simulink model "Engine_Combustion_Model"  (R2016b)
settings: Solver=FixedStepAuto  StartTime=0.0  StopTime=inf  FixedStep=EngMdl.tiSimnTiStep_C  RelTol=1e-3  SampleTimeConstraint=STIndependent  EnableMultiTasking=on
undefined symbols (not defined in the file or in its folder): EngMdl
(part 1 of 2)
settings Model: Creator=m01wolf  LastModifiedBy=bunver
settings DataIOCC: SaveFormat=StructureWithTime  SaveOutput=off  DSMLogging=off  VisualizeSimOutput=off  SaveTime=off  StateSaveName=Results  SignalLoggingName=Results
settings OptimizationCC: BlockReduction=off  ConditionallyExecuteInputs=off  LifeSpan=inf
settings DebuggingCC: AllowSymbolicDim=off  SFUnexpectedBacktrackingDiag=warning  SFNoUnconditionalDefaultTransitionDiag=warning  SFExecutionAtInitializationDiag=none
settings ModelReferenceCC: ModelReferenceNumInstancesAllowed=Single  PropagateSignalLabelsOutOfModel=off
settings GRTTargetCC: TargetLangStandard=C89/C90 (ANSI)
settings ConfigComp: CovMetricSettings=dw  CovHtmlReporting=on  CovSaveCumulativeToWorkspaceVar=on  CovSaveSingleToWorkspaceVar=on  CovExternalEMLEnable=off

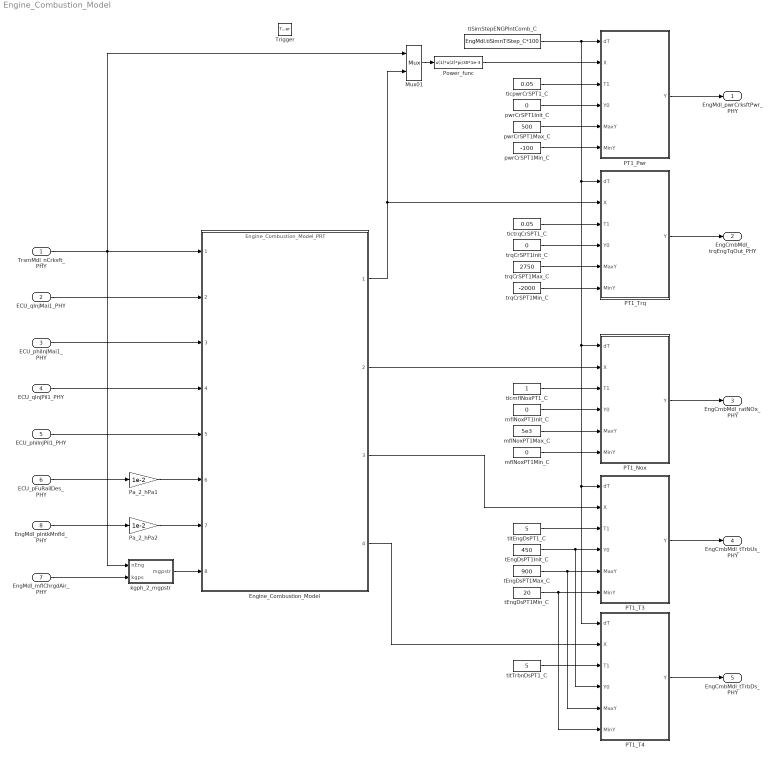
== system Engine_Combustion_Model ==
  TrsmMdl_nCrksft_PHY : Inport
  ECU_qInjMai1_PHY : Inport  Port=2
  ECU_phiInjMai1_PHY : Inport  Port=3
  ECU_qInjPil1_PHY : Inport  Port=4
  ECU_phiInjPil1_PHY : Inport  Port=5
  ECU_pFuRailDes_PHY : Inport  Port=6
  EngMdl_mflChrgdAir_PHY : Inport  Port=7
  EngMdl_pIntkMnfld_PHY : Inport  Port=8
  Trigger : TriggerPort  TriggerType=function-call  VariantControl=Variant  PortDimensions=1
  Engine_Combustion_Model : ModelReference  ModelNameDialog=Engine_Combustion_Model_PRT.slxp  ModelReferenceVersion=1.251  CopyOfModelProtected=on
  Mux01 : Mux  Inputs=2
  PT1_Nox : Subsystem
  PT1_Pwr : Subsystem
  PT1_T3 : Subsystem
  PT1_T4 : Subsystem
  PT1_Trq : Subsystem
  Pa_2_hPa1 : Gain  Gain=1e-2
  Pa_2_hPa2 : Gain  Gain=1e-2
  Power_func : Fcn  Expr=u(1)*u(2)*pi/30*1e-3
  kgph_2_mgpstr : Subsystem
  mflNoxPT1Init_C : Constant  Value=0
  mflNoxPT1Max_C : Constant  Value=5e3
  mflNoxPT1Min_C : Constant  Value=0
  pwrCrSPT1Init_C : Constant  Value=0
  pwrCrSPT1Max_C : Constant  Value=500
  pwrCrSPT1Min_C : Constant  Value=-100
  tEngDsPT1Init_C : Constant  Value=450  SampleTime=-1
  tEngDsPT1Max_C : Constant  Value=900  SampleTime=-1
  tEngDsPT1Min_C : Constant  Value=20  SampleTime=-1
  tiSimStepENGPlntComb_C : Constant  Value=EngMdl.tiSimnTiStep_C*100  SampleTime=-1
  ticmflNoxPT1_C : Constant
  ticpwrCrSPT1_C : Constant  Value=0.05
  tictrqCrSPT1_C : Constant  Value=0.05  SampleTime=-1
  titEngDsPT1_C : Constant  Value=5  SampleTime=-1
  titTrbnDsPT1_C : Constant  Value=5  SampleTime=-1
  trqCrSPT1Init_C : Constant  Value=0  SampleTime=-1
  trqCrSPT1Max_C : Constant  Value=2750  SampleTime=-1
  trqCrSPT1Min_C : Constant  Value=-2000  SampleTime=-1
  EngMdl_pwrCrksftPwr_PHY : Outport
  EngCmbMdl_trqEngTqOut_PHY : Outport  Port=2
  EngCmbMdl_ratNOx_PHY : Outport  Port=3
  EngCmbMdl_tTrbUs_PHY : Outport  Port=4
  EngCmbMdl_tTrbDs_PHY : Outport  Port=5
  wires:
  Pa_2_hPa1/1 -> Engine_Combustion_Model/6
  Pa_2_hPa2/1 -> Engine_Combustion_Model/7
  kgph_2_mgpstr/1(mgpstr) -> Engine_Combustion_Model/8
  ECU_qInjMai1_PHY/1 -> Engine_Combustion_Model/2
  ECU_phiInjMai1_PHY/1 -> Engine_Combustion_Model/3
  ECU_qInjPil1_PHY/1 -> Engine_Combustion_Model/4
  ECU_phiInjPil1_PHY/1 -> Engine_Combustion_Model/5
  ECU_pFuRailDes_PHY/1 -> Pa_2_hPa1/1
  EngMdl_mflChrgdAir_PHY/1 -> kgph_2_mgpstr/2(kgps)
  EngMdl_pIntkMnfld_PHY/1 -> Pa_2_hPa2/1
  Engine_Combustion_Model/1 -> Mux01/2, PT1_Trq/2(X)
  TrsmMdl_nCrksft_PHY/1 -> Mux01/1, Engine_Combustion_Model/1, kgph_2_mgpstr/1(nEng)
  Mux01/1 -> Power_func/1
  Engine_Combustion_Model/2 -> PT1_Nox/2(X)
  tEngDsPT1Init_C/1 -> PT1_T3/4(Y0), PT1_T4/4(Y0)
  tEngDsPT1Max_C/1 -> PT1_T3/5(MaxY), PT1_T4/5(MaxY)
  titEngDsPT1_C/1 -> PT1_T3/3(T1)
  PT1_T3/1(Y) -> EngCmbMdl_tTrbUs_PHY/1
  tEngDsPT1Min_C/1 -> PT1_T3/6(MinY), PT1_T4/6(MinY)
  Engine_Combustion_Model/3 -> PT1_T3/2(X)
  Engine_Combustion_Model/4 -> PT1_T4/2(X)
  titTrbnDsPT1_C/1 -> PT1_T4/3(T1)
  PT1_T4/1(Y) -> EngCmbMdl_tTrbDs_PHY/1
  ticmflNoxPT1_C/1 -> PT1_Nox/3(T1)
  mflNoxPT1Init_C/1 -> PT1_Nox/4(Y0)
  mflNoxPT1Max_C/1 -> PT1_Nox/5(MaxY)
  mflNoxPT1Min_C/1 -> PT1_Nox/6(MinY)
  PT1_Nox/1(Y) -> EngCmbMdl_ratNOx_PHY/1
  tictrqCrSPT1_C/1 -> PT1_Trq/3(T1)
  trqCrSPT1Init_C/1 -> PT1_Trq/4(Y0)
  trqCrSPT1Max_C/1 -> PT1_Trq/5(MaxY)
  trqCrSPT1Min_C/1 -> PT1_Trq/6(MinY)
  PT1_Trq/1(Y) -> EngCmbMdl_trqEngTqOut_PHY/1
  ticpwrCrSPT1_C/1 -> PT1_Pwr/3(T1)
  pwrCrSPT1Init_C/1 -> PT1_Pwr/4(Y0)
  pwrCrSPT1Max_C/1 -> PT1_Pwr/5(MaxY)
  pwrCrSPT1Min_C/1 -> PT1_Pwr/6(MinY)
  PT1_Pwr/1(Y) -> EngMdl_pwrCrksftPwr_PHY/1
  Power_func/1 -> PT1_Pwr/2(X)
  tiSimStepENGPlntComb_C/1 -> PT1_Trq/1(dT), PT1_Nox/1(dT), PT1_T3/1(dT), PT1_T4/1(dT), PT1_Pwr/1(dT)

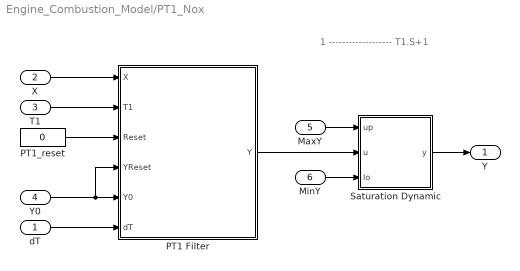
== system Engine_Combustion_Model/PT1_Nox ==
  note: 1
      | -------------------
      | T1.S+1
  dT : Inport
  X : Inport  Port=2
  T1 : Inport  Port=3
  Y0 : Inport  Port=4
  MaxY : Inport  Port=5
  MinY : Inport  Port=6
  PT1 Filter : Subsystem  mask(PT1 Filter){}
      mask help:
      | Proportional filter with first order time constant, unit gain and external reset.
      |
      | X: Input value
      | T1: Time constant of proportional filter
      | Reset: Reset status
      | YReset: Output value during reset
      | Y0: Initial value of output
      | Y: Output value
      | dT: Sample time
      mask Display:
      | color('blue');
      | fprintf('PT1\nFilter');
      | 
      | color('black');
      | port_label('input', 1, 'X');
      | port_label('input', 2, 'T1');
      | port_label('input', 3, 'Reset');
      | port_label('input', 4, 'YReset');
      | port_label('input', 5, 'Y0');
      | port_label('input', 6, 'dT');
      | port_label('output', 1, 'Y');
  PT1_reset : Constant  Value=0  SampleTime=-1
  Saturation Dynamic : Subsystem  mask(Saturation Dynamic){OutMin=[], OutMax=[], OutDataTypeStr=Inherit: Same as second input, OutputDataTypeScalingMode=Same as second input, OutDataType=fixdt(1, 16), OutScaling=2^-10, LockScale=off, RndMeth=Floor, DoSatur=off}
      mask prompts: OutMin "Simulink:masks:OutputMinimum_MP"; OutMax "Simulink:masks:OutputMaximum_MP"; OutDataTypeStr "Simulink:masks:OutputDataType_MP"; OutputDataTypeScalingMode "Simulink:masks:OutputDataTypeMode_MP"; OutDataType "Simulink:masks:OutputDataTypeegFixdt116Fixdtsingle_MP"; OutScaling "Simulink:masks:OutputScalingSlopeEg29OrSlopeBias_MP"; LockScale "Simulink:masks:LockOutputDataTypeAgainstFxpTools_MP"; RndMeth "Simulink:masks:IntegerRoundingMode_MP"; DoSatur "Simulink:masks:SaturateOnIntegerOverflow_MP"
      mask help: Simulink:masks:SaturationDynamic_MD
      mask init:
      | blkH = gcbh;
      | blkName = getfullname(blkH);
      | 
      | switch_blks = {'Switch','Switch2'}; 
      | for i = 1:length(switch_blks)
      |   set_param([blkName,'/',switch_blks{i}], ...
      |       'RndMeth', RndMeth, ...
      | 	  'DoSatur', DoSatur);
      | end
      | 
      | propBlk = [blkName, '/Data Type Propagation'];
      | 
      | if strcmp(OutputDataTypeScalingMode, 'Same as second input')
      |     set_param(propBlk, 'PropDataTypeMode', 'Inherit via propagation rule', ...
      |                        'PropScalingMode',  'Inherit via propagation rule');
      | else
      |     scaling = OutScaling;
      |     scalingMode = 'Specify via dialog';
      |     switch OutputDataTypeScalingMode
      |       case 'double'
      |         dataType = 'fixdt(''double'')';
      |       case 'single'
      |         dataType = 'fixdt(''single'')';
      |       case 'int8'
      |         dataType = 'fixdt(1,8,0)';
      |       case 'uint8'
      |         dataType = 'fixdt(0,8,0)';
      |       case 'int16'
      |         dataType = 'fixdt(1,16,0)';
      |       case 'uint16'
      |         dataType = 'fixdt(0,16,0)';
      |       case 'int32'
      |         dataType = 'fixdt(1,32,0)';
      |       case 'uint32'
      |         dataType = 'fixdt(0,32,0)';
      |       case 'Specify via dialog'
      |         dataType = OutDataType;
      |         if ~isempty(OutDataTypeStr) && isa(OutDataTypeStr,'Simulink.NumericType') 
      |           if strcmp(OutDataTypeStr.DataTypeMode, 'Fixed-point: unspecified scaling') 
      |             scalingMode = 'Obtain via best precision';
      |             range = [OutMin OutMax];
      |             range = range(~isinf(range));
      |             set_param(propBlk, 'ValuesUsedBestPrec', mat2str(range));
      |           end
      |         end
      |     end
      |     
      |     set_param(propBlk, 'PropDataTypeMode', 'Specify via dialog', ...
      |                        'PropScalingMode',  scalingMode, ...
      |                        'PropDataType',     dataType, ...
      |                        'PropScaling',      scaling);
      | end
      mask Callback OutDataTypeStr: fixptdialog(gcbh)
      mask TypeOptions OutputDataTypeScalingMode: double | single | int8 | uint8 | int16 | uint16 | int32 | uint32 | Specify via dialog | Same as second input
      mask Callback OutputDataTypeScalingMode: fixptdialog(gcbh)
      mask Callback OutDataType: fixptdialog(gcbh)
      mask TypeOptions RndMeth: Simulink:masks:Ceiling | Simulink:masks:Convergent | Simulink:masks:Floor | Simulink:masks:Nearest | Simulink:masks:Round | Simulink:masks:Simplest | Simulink:masks:Zero
  Y : Outport
  wires:
  dT/1 -> PT1 Filter/6(dT)
  MaxY/1 -> Saturation Dynamic/1(up)
  T1/1 -> PT1 Filter/2(T1)
  X/1 -> PT1 Filter/1(X)
  MinY/1 -> Saturation Dynamic/3(lo)
  Y0/1 -> PT1 Filter/5(Y0), PT1 Filter/4(YReset)
  Saturation Dynamic/1(y) -> Y/1
  PT1 Filter/1(Y) -> Saturation Dynamic/2(u)
  PT1_reset/1 -> PT1 Filter/3(Reset)

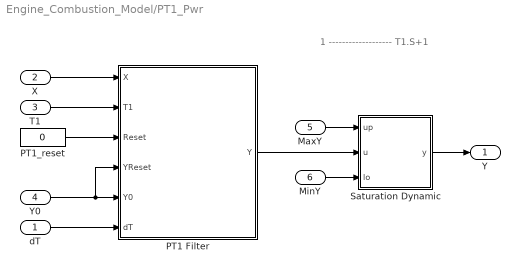
== system Engine_Combustion_Model/PT1_Pwr ==
  note: 1
      | -------------------
      | T1.S+1
  dT : Inport
  X : Inport  Port=2
  T1 : Inport  Port=3
  Y0 : Inport  Port=4
  MaxY : Inport  Port=5
  MinY : Inport  Port=6
  PT1 Filter : Subsystem  mask(PT1 Filter){}
      mask help:
      | Proportional filter with first order time constant, unit gain and external reset.
      |
      | X: Input value
      | T1: Time constant of proportional filter
      | Reset: Reset status
      | YReset: Output value during reset
      | Y0: Initial value of output
      | Y: Output value
      | dT: Sample time
      mask Display:
      | color('blue');
      | fprintf('PT1\nFilter');
      | 
      | color('black');
      | port_label('input', 1, 'X');
      | port_label('input', 2, 'T1');
      | port_label('input', 3, 'Reset');
      | port_label('input', 4, 'YReset');
      | port_label('input', 5, 'Y0');
      | port_label('input', 6, 'dT');
      | port_label('output', 1, 'Y');
  PT1_reset : Constant  Value=0  SampleTime=-1
  Saturation Dynamic : Subsystem  mask(Saturation Dynamic){OutMin=[], OutMax=[], OutDataTypeStr=Inherit: Same as second input, OutputDataTypeScalingMode=Same as second input, OutDataType=fixdt(1, 16), OutScaling=2^-10, LockScale=off, RndMeth=Floor, DoSatur=off}
      mask prompts: OutMin "Simulink:masks:OutputMinimum_MP"; OutMax "Simulink:masks:OutputMaximum_MP"; OutDataTypeStr "Simulink:masks:OutputDataType_MP"; OutputDataTypeScalingMode "Simulink:masks:OutputDataTypeMode_MP"; OutDataType "Simulink:masks:OutputDataTypeegFixdt116Fixdtsingle_MP"; OutScaling "Simulink:masks:OutputScalingSlopeEg29OrSlopeBias_MP"; LockScale "Simulink:masks:LockOutputDataTypeAgainstFxpTools_MP"; RndMeth "Simulink:masks:IntegerRoundingMode_MP"; DoSatur "Simulink:masks:SaturateOnIntegerOverflow_MP"
      mask help: Simulink:masks:SaturationDynamic_MD
      mask init: same as Engine_Combustion_Model/PT1_Nox/Saturation Dynamic
      mask Callback OutDataTypeStr: fixptdialog(gcbh)
      mask TypeOptions OutputDataTypeScalingMode: double | single | int8 | uint8 | int16 | uint16 | int32 | uint32 | Specify via dialog | Same as second input
      mask Callback OutputDataTypeScalingMode: fixptdialog(gcbh)
      mask Callback OutDataType: fixptdialog(gcbh)
      mask TypeOptions RndMeth: Simulink:masks:Ceiling | Simulink:masks:Convergent | Simulink:masks:Floor | Simulink:masks:Nearest | Simulink:masks:Round | Simulink:masks:Simplest | Simulink:masks:Zero
  Y : Outport
  wires:
  dT/1 -> PT1 Filter/6(dT)
  MaxY/1 -> Saturation Dynamic/1(up)
  T1/1 -> PT1 Filter/2(T1)
  X/1 -> PT1 Filter/1(X)
  MinY/1 -> Saturation Dynamic/3(lo)
  Y0/1 -> PT1 Filter/5(Y0), PT1 Filter/4(YReset)
  Saturation Dynamic/1(y) -> Y/1
  PT1 Filter/1(Y) -> Saturation Dynamic/2(u)
  PT1_reset/1 -> PT1 Filter/3(Reset)

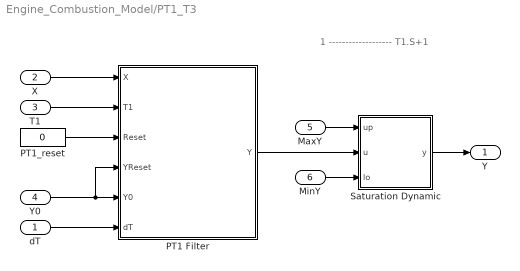
== system Engine_Combustion_Model/PT1_T3 ==
  note: 1
      | -------------------
      | T1.S+1
  dT : Inport
  X : Inport  Port=2
  T1 : Inport  Port=3
  Y0 : Inport  Port=4
  MaxY : Inport  Port=5
  MinY : Inport  Port=6
  PT1 Filter : Subsystem  mask(PT1 Filter){}
      mask help:
      | Proportional filter with first order time constant, unit gain and external reset.
      |
      | X: Input value
      | T1: Time constant of proportional filter
      | Reset: Reset status
      | YReset: Output value during reset
      | Y0: Initial value of output
      | Y: Output value
      | dT: Sample time
      mask Display:
      | color('blue');
      | fprintf('PT1\nFilter');
      | 
      | color('black');
      | port_label('input', 1, 'X');
      | port_label('input', 2, 'T1');
      | port_label('input', 3, 'Reset');
      | port_label('input', 4, 'YReset');
      | port_label('input', 5, 'Y0');
      | port_label('input', 6, 'dT');
      | port_label('output', 1, 'Y');
  PT1_reset : Constant  Value=0  SampleTime=-1
  Saturation Dynamic : Subsystem  mask(Saturation Dynamic){OutMin=[], OutMax=[], OutDataTypeStr=Inherit: Same as second input, OutputDataTypeScalingMode=Same as second input, OutDataType=fixdt(1, 16), OutScaling=2^-10, LockScale=off, RndMeth=Floor, DoSatur=off}
      mask prompts: OutMin "Simulink:masks:OutputMinimum_MP"; OutMax "Simulink:masks:OutputMaximum_MP"; OutDataTypeStr "Simulink:masks:OutputDataType_MP"; OutputDataTypeScalingMode "Simulink:masks:OutputDataTypeMode_MP"; OutDataType "Simulink:masks:OutputDataTypeegFixdt116Fixdtsingle_MP"; OutScaling "Simulink:masks:OutputScalingSlopeEg29OrSlopeBias_MP"; LockScale "Simulink:masks:LockOutputDataTypeAgainstFxpTools_MP"; RndMeth "Simulink:masks:IntegerRoundingMode_MP"; DoSatur "Simulink:masks:SaturateOnIntegerOverflow_MP"
      mask help: Simulink:masks:SaturationDynamic_MD
      mask init: same as Engine_Combustion_Model/PT1_Nox/Saturation Dynamic
      mask Callback OutDataTypeStr: fixptdialog(gcbh)
      mask TypeOptions OutputDataTypeScalingMode: double | single | int8 | uint8 | int16 | uint16 | int32 | uint32 | Specify via dialog | Same as second input
      mask Callback OutputDataTypeScalingMode: fixptdialog(gcbh)
      mask Callback OutDataType: fixptdialog(gcbh)
      mask TypeOptions RndMeth: Simulink:masks:Ceiling | Simulink:masks:Convergent | Simulink:masks:Floor | Simulink:masks:Nearest | Simulink:masks:Round | Simulink:masks:Simplest | Simulink:masks:Zero
  Y : Outport
  wires:
  PT1_reset/1 -> PT1 Filter/3(Reset)
  PT1 Filter/1(Y) -> Saturation Dynamic/2(u)
  Saturation Dynamic/1(y) -> Y/1
  Y0/1 -> PT1 Filter/4(YReset), PT1 Filter/5(Y0)
  MinY/1 -> Saturation Dynamic/3(lo)
  X/1 -> PT1 Filter/1(X)
  T1/1 -> PT1 Filter/2(T1)
  MaxY/1 -> Saturation Dynamic/1(up)
  dT/1 -> PT1 Filter/6(dT)

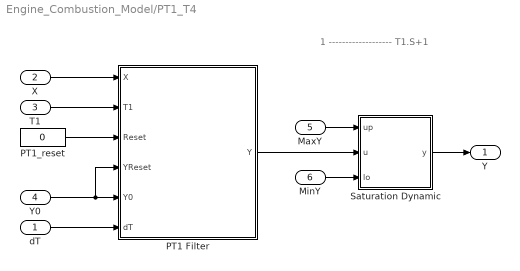
== system Engine_Combustion_Model/PT1_T4 ==
  note: 1
      | -------------------
      | T1.S+1
  dT : Inport
  X : Inport  Port=2
  T1 : Inport  Port=3
  Y0 : Inport  Port=4
  MaxY : Inport  Port=5
  MinY : Inport  Port=6
  PT1 Filter : Subsystem  mask(PT1 Filter){}
      mask help:
      | Proportional filter with first order time constant, unit gain and external reset.
      |
      | X: Input value
      | T1: Time constant of proportional filter
      | Reset: Reset status
      | YReset: Output value during reset
      | Y0: Initial value of output
      | Y: Output value
      | dT: Sample time
      mask Display:
      | color('blue');
      | fprintf('PT1\nFilter');
      | 
      | color('black');
      | port_label('input', 1, 'X');
      | port_label('input', 2, 'T1');
      | port_label('input', 3, 'Reset');
      | port_label('input', 4, 'YReset');
      | port_label('input', 5, 'Y0');
      | port_label('input', 6, 'dT');
      | port_label('output', 1, 'Y');
  PT1_reset : Constant  Value=0  SampleTime=-1
  Saturation Dynamic : Subsystem  mask(Saturation Dynamic){OutMin=[], OutMax=[], OutDataTypeStr=Inherit: Same as second input, OutputDataTypeScalingMode=Same as second input, OutDataType=fixdt(1, 16), OutScaling=2^-10, LockScale=off, RndMeth=Floor, DoSatur=off}
      mask prompts: OutMin "Simulink:masks:OutputMinimum_MP"; OutMax "Simulink:masks:OutputMaximum_MP"; OutDataTypeStr "Simulink:masks:OutputDataType_MP"; OutputDataTypeScalingMode "Simulink:masks:OutputDataTypeMode_MP"; OutDataType "Simulink:masks:OutputDataTypeegFixdt116Fixdtsingle_MP"; OutScaling "Simulink:masks:OutputScalingSlopeEg29OrSlopeBias_MP"; LockScale "Simulink:masks:LockOutputDataTypeAgainstFxpTools_MP"; RndMeth "Simulink:masks:IntegerRoundingMode_MP"; DoSatur "Simulink:masks:SaturateOnIntegerOverflow_MP"
      mask help: Simulink:masks:SaturationDynamic_MD
      mask init: same as Engine_Combustion_Model/PT1_Nox/Saturation Dynamic
      mask Callback OutDataTypeStr: fixptdialog(gcbh)
      mask TypeOptions OutputDataTypeScalingMode: double | single | int8 | uint8 | int16 | uint16 | int32 | uint32 | Specify via dialog | Same as second input
      mask Callback OutputDataTypeScalingMode: fixptdialog(gcbh)
      mask Callback OutDataType: fixptdialog(gcbh)
      mask TypeOptions RndMeth: Simulink:masks:Ceiling | Simulink:masks:Convergent | Simulink:masks:Floor | Simulink:masks:Nearest | Simulink:masks:Round | Simulink:masks:Simplest | Simulink:masks:Zero
  Y : Outport
  wires:
  dT/1 -> PT1 Filter/6(dT)
  MaxY/1 -> Saturation Dynamic/1(up)
  T1/1 -> PT1 Filter/2(T1)
  X/1 -> PT1 Filter/1(X)
  MinY/1 -> Saturation Dynamic/3(lo)
  Y0/1 -> PT1 Filter/5(Y0), PT1 Filter/4(YReset)
  Saturation Dynamic/1(y) -> Y/1
  PT1 Filter/1(Y) -> Saturation Dynamic/2(u)
  PT1_reset/1 -> PT1 Filter/3(Reset)

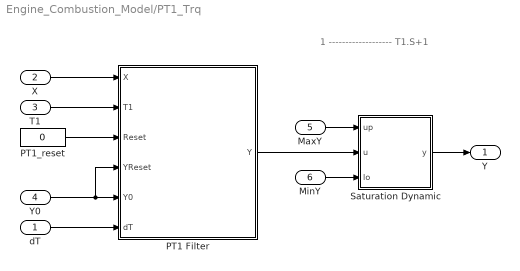
== system Engine_Combustion_Model/PT1_Trq ==
  note: 1
      | -------------------
      | T1.S+1
  dT : Inport
  X : Inport  Port=2
  T1 : Inport  Port=3
  Y0 : Inport  Port=4
  MaxY : Inport  Port=5
  MinY : Inport  Port=6
  PT1 Filter : Subsystem  mask(PT1 Filter){}
      mask help:
      | Proportional filter with first order time constant, unit gain and external reset.
      |
      | X: Input value
      | T1: Time constant of proportional filter
      | Reset: Reset status
      | YReset: Output value during reset
      | Y0: Initial value of output
      | Y: Output value
      | dT: Sample time
      mask Display:
      | color('blue');
      | fprintf('PT1\nFilter');
      | 
      | color('black');
      | port_label('input', 1, 'X');
      | port_label('input', 2, 'T1');
      | port_label('input', 3, 'Reset');
      | port_label('input', 4, 'YReset');
      | port_label('input', 5, 'Y0');
      | port_label('input', 6, 'dT');
      | port_label('output', 1, 'Y');
  PT1_reset : Constant  Value=0  SampleTime=-1
  Saturation Dynamic : Subsystem  mask(Saturation Dynamic){OutMin=[], OutMax=[], OutDataTypeStr=Inherit: Same as second input, OutputDataTypeScalingMode=Same as second input, OutDataType=fixdt(1, 16), OutScaling=2^-10, LockScale=off, RndMeth=Floor, DoSatur=off}
      mask prompts: OutMin "Simulink:masks:OutputMinimum_MP"; OutMax "Simulink:masks:OutputMaximum_MP"; OutDataTypeStr "Simulink:masks:OutputDataType_MP"; OutputDataTypeScalingMode "Simulink:masks:OutputDataTypeMode_MP"; OutDataType "Simulink:masks:OutputDataTypeegFixdt116Fixdtsingle_MP"; OutScaling "Simulink:masks:OutputScalingSlopeEg29OrSlopeBias_MP"; LockScale "Simulink:masks:LockOutputDataTypeAgainstFxpTools_MP"; RndMeth "Simulink:masks:IntegerRoundingMode_MP"; DoSatur "Simulink:masks:SaturateOnIntegerOverflow_MP"
      mask help: Simulink:masks:SaturationDynamic_MD
      mask init: same as Engine_Combustion_Model/PT1_Nox/Saturation Dynamic
      mask Callback OutDataTypeStr: fixptdialog(gcbh)
      mask TypeOptions OutputDataTypeScalingMode: double | single | int8 | uint8 | int16 | uint16 | int32 | uint32 | Specify via dialog | Same as second input
      mask Callback OutputDataTypeScalingMode: fixptdialog(gcbh)
      mask Callback OutDataType: fixptdialog(gcbh)
      mask TypeOptions RndMeth: Simulink:masks:Ceiling | Simulink:masks:Convergent | Simulink:masks:Floor | Simulink:masks:Nearest | Simulink:masks:Round | Simulink:masks:Simplest | Simulink:masks:Zero
  Y : Outport
  wires:
  PT1_reset/1 -> PT1 Filter/3(Reset)
  PT1 Filter/1(Y) -> Saturation Dynamic/2(u)
  Saturation Dynamic/1(y) -> Y/1
  Y0/1 -> PT1 Filter/4(YReset), PT1 Filter/5(Y0)
  MinY/1 -> Saturation Dynamic/3(lo)
  X/1 -> PT1 Filter/1(X)
  T1/1 -> PT1 Filter/2(T1)
  MaxY/1 -> Saturation Dynamic/1(up)
  dT/1 -> PT1 Filter/6(dT)

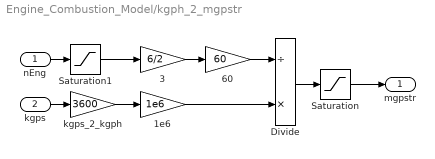
== system Engine_Combustion_Model/kgph_2_mgpstr ==
  nEng : Inport
  kgps : Inport  Port=2
  1e6 : Gain  Gain=1e6
  3 : Gain  Gain=6/2
  60 : Gain  Gain=60
  Divide : Product  Inputs=/*
  Saturation : Saturate  UpperLimit=inf  LowerLimit=0
  Saturation1 : Saturate  UpperLimit=inf  LowerLimit=300
  kgps_2_kgph : Gain  Gain=3600
  mgpstr : Outport
  wires:
  Saturation1/1 -> 3/1
  Divide/1 -> Saturation/1
  nEng/1 -> Saturation1/1
  kgps/1 -> kgps_2_kgph/1
  Saturation/1 -> mgpstr/1
  kgps_2_kgph/1 -> 1e6/1
  1e6/1 -> Divide/2
  3/1 -> 60/1
  60/1 -> Divide/1

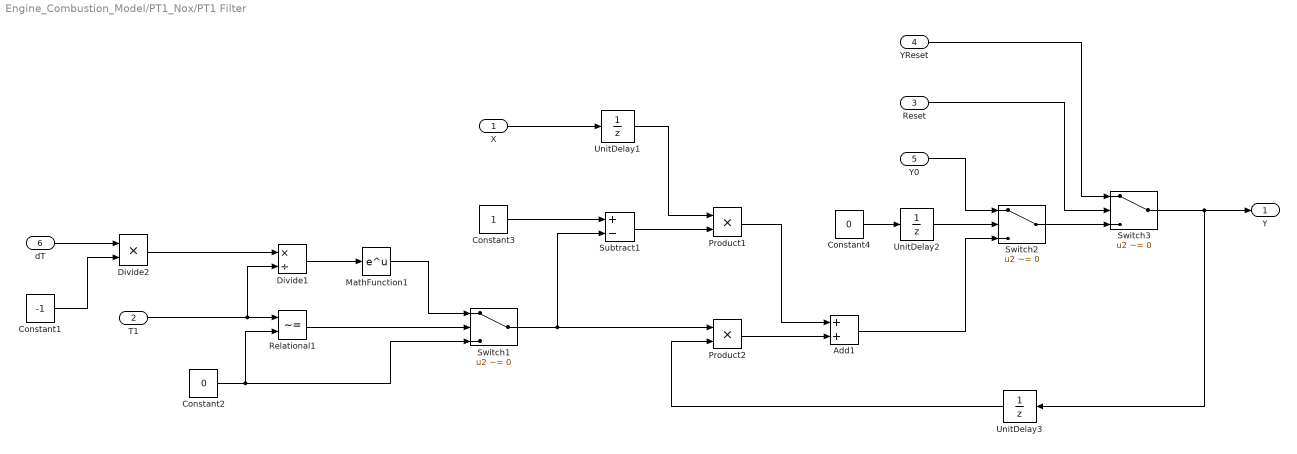
== system Engine_Combustion_Model/PT1_Nox/PT1 Filter ==
  X : Inport
  T1 : Inport  Port=2
  Reset : Inport  Port=3
  YReset : Inport  Port=4
  Y0 : Inport  Port=5
  dT : Inport  Port=6
  Add1 : Sum
  Constant1 : Constant  Value=-1
  Constant2 : Constant  Value=0
  Constant3 : Constant
  Constant4 : Constant  Value=0
  Divide1 : Product  Inputs=*/
  Divide2 : Product  Inputs=**
  MathFunction1 : Math  SaturateOnIntegerOverflow=on
  Product1 : Product  RndMeth=Zero
  Product2 : Product  RndMeth=Zero
  Relational1 : RelationalOperator  Operator=~=  OutDataTypeStr=boolean  RndMeth=Nearest
  Subtract1 : Sum  Inputs=+-
  Switch1 : Switch  Criteria=u2 ~= 0
  Switch2 : Switch  Criteria=u2 ~= 0
  Switch3 : Switch  Criteria=u2 ~= 0
  UnitDelay1 : UnitDelay  SampleTime=-1
  UnitDelay2 : UnitDelay  InitialCondition=1  SampleTime=-1
  UnitDelay3 : UnitDelay  SampleTime=-1
  Y : Outport
  wires:
  dT/1 -> Divide2/1
  Constant2/1 -> Relational1/2, Switch1/3
  MathFunction1/1 -> Switch1/1
  Relational1/1 -> Switch1/2
  Switch2/1 -> Switch3/3
  Add1/1 -> Switch2/3
  Switch3/1 -> Y/1, UnitDelay3/1
  Y0/1 -> Switch2/1
  UnitDelay2/1 -> Switch2/2
  Constant4/1 -> UnitDelay2/1
  YReset/1 -> Switch3/1
  Reset/1 -> Switch3/2
  UnitDelay3/1 -> Product2/2
  Switch1/1 -> Product2/1, Subtract1/2
  Product2/1 -> Add1/2
  Product1/1 -> Add1/1
  Subtract1/1 -> Product1/2
  UnitDelay1/1 -> Product1/1
  X/1 -> UnitDelay1/1
  Constant3/1 -> Subtract1/1
  Divide1/1 -> MathFunction1/1
  Divide2/1 -> Divide1/1
  T1/1 -> Relational1/1, Divide1/2
  Constant1/1 -> Divide2/2

== system Engine_Combustion_Model/PT1_Nox/Saturation Dynamic ==
  up : Inport
  u : Inport  Port=2
  lo : Inport  Port=3
  Data Type Duplicate : DataTypeDuplicate  DisableCoverage=on
  Data Type Propagation : S-Function  FunctionName=sfix_dtprop  Parameters=14,PropDataTypeMode,(getdatatypespecs(PropDataType,PropScaling,DblOver,0, 0, PropDataTypeMode, PropScalingMode)),IfRefDouble,IfRefSingle,IsSigned,NumBitsBase,NumBitsMult,NumBitsAdd,(sort(reshape(round(NumBitsAllowFinal), prod(size(NumBitsAllowFinal)),1))),PropScalingMode,ValuesUsedBestPrec,SlopeBase,SlopeMult,SlopeAdd,BiasBase,BiasMult,BiasAdd,DblOver  SFunctionDeploymentMode=off  EnableBusSupport=off  mask(Data Type Propagation){PropDataTypeMode=Inherit via propagation rule, PropDataType=fixdt(1, 16), IfRefDouble=double, IfRefSingle=single, IsSigned=IsSigned1, NumBitsBase=NumBits1, NumBitsMult=1, NumBitsAdd=0, NumBitsAllowFinal=1:128, PropScalingMode=Inherit via propagation rule, PropScaling=2^-10, ValuesUsedBestPrec=[5 -7], SlopeBase=Slope1, SlopeMult=1, SlopeAdd=0, BiasBase=Bias1, BiasMult=1, BiasAdd=0}
      mask prompts: PropDataTypeMode "Simulink:masks:x1PropagatedDataType_MP"; PropDataType "Simulink:masks:x11PropagatedDataTypeegFixdt116Fixdtsingle_MP"; IfRefDouble "Simulink:masks:x11IfAnyReferenceInputIsDoubleOutputIs_MP"; IfRefSingle "Simulink:masks:x12IfAnyReferenceInputIsSingleOutputIs_MP"; IsSigned "Simulink:masks:x13IsSigned_MP"; NumBitsBase "Simulink:masks:x141NumberofBitsBase_MP"; NumBitsMult "Simulink:masks:x142NumberofBitsMultiplicativeAdjustment_MP"; NumBitsAdd "Simulink:masks:x143NumberofBitsAdditiveAdjustment_MP"; NumBitsAllowFinal "Simulink:masks:x144NumberofBitsAllowableFinalValues_MP"; PropScalingMode "Simulink:masks:x2PropagatedScaling_MP"; PropScaling "Simulink:masks:x21PropagatedScalingSlopeEg29OrSlopeBiasEg1253_MP"; ValuesUsedBestPrec "Simulink:masks:x21ValuesUsedToDetermineBestPrecisionScaling_MP"; SlopeBase "Simulink:masks:x211SlopeBase_MP"; SlopeMult "Simulink:masks:x212SlopeMultiplicativeAdjustment_MP"; SlopeAdd "Simulink:masks:x213SlopeAdditiveAdjustment_MP"; BiasBase "Simulink:masks:x221BiasBase_MP"; BiasMult "Simulink:masks:x222BiasMultiplicativeAdjustment_MP"; BiasAdd "Simulink:masks:x223BiasAdditiveAdjustment_MP"
      mask help: Simulink:masks:DataTypePropagation_MD
      mask init:
      | DblOver = 0;
      mask TypeOptions PropDataTypeMode: Simulink:masks:SpecifyViaDialog | Simulink:masks:InheritViaPropagationRule
      mask Callback PropDataTypeMode: fixptdialog(gcbh)
      mask Callback PropDataType: fixptdialog(gcbh)
      mask TypeOptions IfRefDouble: Simulink:masks:double | Simulink:masks:single
      mask TypeOptions IfRefSingle: Simulink:masks:double | Simulink:masks:single
      mask TypeOptions IsSigned: Simulink:masks:IsSigned1 | Simulink:masks:IsSigned2 | Simulink:masks:IsSigned1OrIsSigned2 | Simulink:masks:TRUE | Simulink:masks:FALSE
      mask TypeOptions NumBitsBase: NumBits1 | NumBits2 | max([NumBits1 NumBits2]) | min([NumBits1 NumBits2]) | NumBits1+NumBits2
      mask TypeOptions PropScalingMode: Simulink:masks:SpecifyViaDialog | Simulink:masks:InheritViaPropagationRule | Simulink:masks:ObtainViaBestPrecision
      mask Callback PropScalingMode: fixptdialog(gcbh)
      mask TypeOptions SlopeBase: Slope1 | Slope2 | max([Slope1 Slope2]) | min([Slope1 Slope2]) | Slope1*Slope2 | Slope1/Slope2 | PosRange1 | PosRange2 | max([PosRange1 PosRange2]) | min([PosRange1 PosRange2]) | PosRange1*PosRange2 | PosRange1/PosRange2
      mask TypeOptions BiasBase: Bias1 | Bias2 | max([Bias1 Bias2]) | min([Bias1 Bias2]) | Bias1*Bias2 | Bias1/Bias2 | Bias1+Bias2 | Bias1-Bias2
      mask Display:
      | port_label('Input',1,'Ref1');
      | port_label('Input',2,'Ref2');
      | port_label('Input',3,'Prop');
  LowerRelop1 : RelationalOperator  DisableCoverage=on  Operator=>  OutDataTypeStr=boolean  RndMeth=Nearest
  Switch : Switch  Criteria=u2 ~= 0  OutDataTypeStr=Inherit: Inherit via back propagation  ZeroCross=off
  Switch2 : Switch  Criteria=u2 ~= 0  OutMin=OutMin  OutMax=OutMax  OutDataTypeStr=Inherit: Inherit via back propagation  ZeroCross=off
  UpperRelop : RelationalOperator  DisableCoverage=on  Operator=<  OutDataTypeStr=boolean  RndMeth=Nearest
  y : Outport  OutMin=OutMin  OutMax=OutMax
  wires:
  up/1 -> Switch2/1, LowerRelop1/2
  u/1 -> Data Type Propagation/2, Data Type Propagation/1, LowerRelop1/1, Switch/3, UpperRelop/1
  lo/1 -> Switch/1, UpperRelop/2
  Switch/1 -> Data Type Duplicate/2, Switch2/3, Data Type Propagation/3
  Switch2/1 -> Data Type Duplicate/1, y/1
  LowerRelop1/1 -> Switch2/2
  UpperRelop/1 -> Switch/2

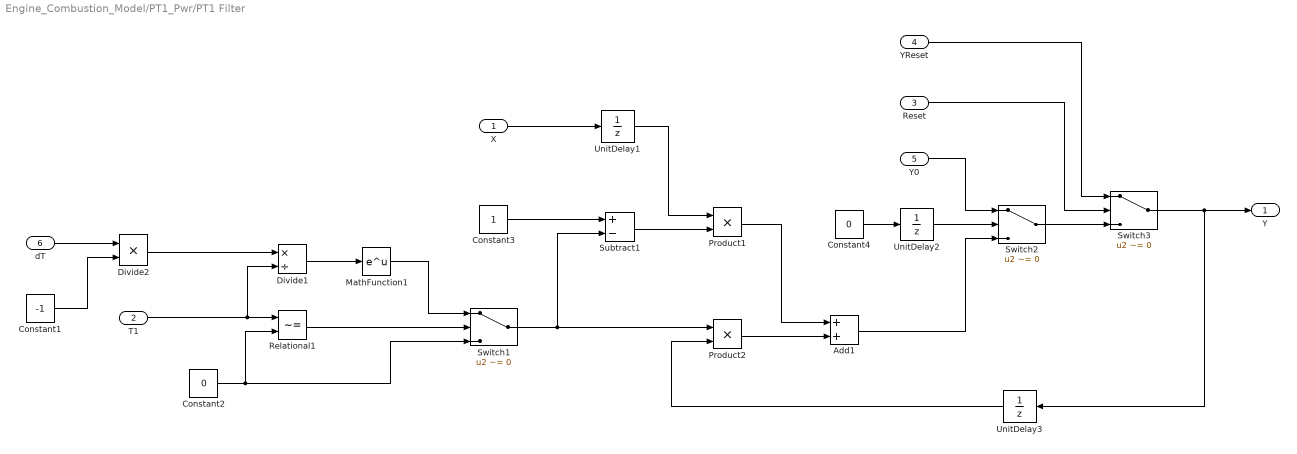
== system Engine_Combustion_Model/PT1_Pwr/PT1 Filter ==
  X : Inport
  T1 : Inport  Port=2
  Reset : Inport  Port=3
  YReset : Inport  Port=4
  Y0 : Inport  Port=5
  dT : Inport  Port=6
  Add1 : Sum
  Constant1 : Constant  Value=-1
  Constant2 : Constant  Value=0
  Constant3 : Constant
  Constant4 : Constant  Value=0
  Divide1 : Product  Inputs=*/
  Divide2 : Product  Inputs=**
  MathFunction1 : Math  SaturateOnIntegerOverflow=on
  Product1 : Product  RndMeth=Zero
  Product2 : Product  RndMeth=Zero
  Relational1 : RelationalOperator  Operator=~=  OutDataTypeStr=boolean  RndMeth=Nearest
  Subtract1 : Sum  Inputs=+-
  Switch1 : Switch  Criteria=u2 ~= 0
  Switch2 : Switch  Criteria=u2 ~= 0
  Switch3 : Switch  Criteria=u2 ~= 0
  UnitDelay1 : UnitDelay  SampleTime=-1
  UnitDelay2 : UnitDelay  InitialCondition=1  SampleTime=-1
  UnitDelay3 : UnitDelay  SampleTime=-1
  Y : Outport
  wires:
  dT/1 -> Divide2/1
  Constant2/1 -> Relational1/2, Switch1/3
  MathFunction1/1 -> Switch1/1
  Relational1/1 -> Switch1/2
  Switch2/1 -> Switch3/3
  Add1/1 -> Switch2/3
  Switch3/1 -> Y/1, UnitDelay3/1
  Y0/1 -> Switch2/1
  UnitDelay2/1 -> Switch2/2
  Constant4/1 -> UnitDelay2/1
  YReset/1 -> Switch3/1
  Reset/1 -> Switch3/2
  UnitDelay3/1 -> Product2/2
  Switch1/1 -> Product2/1, Subtract1/2
  Product2/1 -> Add1/2
  Product1/1 -> Add1/1
  Subtract1/1 -> Product1/2
  UnitDelay1/1 -> Product1/1
  X/1 -> UnitDelay1/1
  Constant3/1 -> Subtract1/1
  Divide1/1 -> MathFunction1/1
  Divide2/1 -> Divide1/1
  T1/1 -> Relational1/1, Divide1/2
  Constant1/1 -> Divide2/2

== system Engine_Combustion_Model/PT1_Pwr/Saturation Dynamic ==
  up : Inport
  u : Inport  Port=2
  lo : Inport  Port=3
  Data Type Duplicate : DataTypeDuplicate  DisableCoverage=on
  Data Type Propagation : S-Function  FunctionName=sfix_dtprop  Parameters=14,PropDataTypeMode,(getdatatypespecs(PropDataType,PropScaling,DblOver,0, 0, PropDataTypeMode, PropScalingMode)),IfRefDouble,IfRefSingle,IsSigned,NumBitsBase,NumBitsMult,NumBitsAdd,(sort(reshape(round(NumBitsAllowFinal), prod(size(NumBitsAllowFinal)),1))),PropScalingMode,ValuesUsedBestPrec,SlopeBase,SlopeMult,SlopeAdd,BiasBase,BiasMult,BiasAdd,DblOver  SFunctionDeploymentMode=off  EnableBusSupport=off  mask(Data Type Propagation){PropDataTypeMode=Inherit via propagation rule, PropDataType=fixdt(1, 16), IfRefDouble=double, IfRefSingle=single, IsSigned=IsSigned1, NumBitsBase=NumBits1, NumBitsMult=1, NumBitsAdd=0, NumBitsAllowFinal=1:128, PropScalingMode=Inherit via propagation rule, PropScaling=2^-10, ValuesUsedBestPrec=[5 -7], SlopeBase=Slope1, SlopeMult=1, SlopeAdd=0, BiasBase=Bias1, BiasMult=1, BiasAdd=0}
      mask prompts: PropDataTypeMode "Simulink:masks:x1PropagatedDataType_MP"; PropDataType "Simulink:masks:x11PropagatedDataTypeegFixdt116Fixdtsingle_MP"; IfRefDouble "Simulink:masks:x11IfAnyReferenceInputIsDoubleOutputIs_MP"; IfRefSingle "Simulink:masks:x12IfAnyReferenceInputIsSingleOutputIs_MP"; IsSigned "Simulink:masks:x13IsSigned_MP"; NumBitsBase "Simulink:masks:x141NumberofBitsBase_MP"; NumBitsMult "Simulink:masks:x142NumberofBitsMultiplicativeAdjustment_MP"; NumBitsAdd "Simulink:masks:x143NumberofBitsAdditiveAdjustment_MP"; NumBitsAllowFinal "Simulink:masks:x144NumberofBitsAllowableFinalValues_MP"; PropScalingMode "Simulink:masks:x2PropagatedScaling_MP"; PropScaling "Simulink:masks:x21PropagatedScalingSlopeEg29OrSlopeBiasEg1253_MP"; ValuesUsedBestPrec "Simulink:masks:x21ValuesUsedToDetermineBestPrecisionScaling_MP"; SlopeBase "Simulink:masks:x211SlopeBase_MP"; SlopeMult "Simulink:masks:x212SlopeMultiplicativeAdjustment_MP"; SlopeAdd "Simulink:masks:x213SlopeAdditiveAdjustment_MP"; BiasBase "Simulink:masks:x221BiasBase_MP"; BiasMult "Simulink:masks:x222BiasMultiplicativeAdjustment_MP"; BiasAdd "Simulink:masks:x223BiasAdditiveAdjustment_MP"
      mask help: Simulink:masks:DataTypePropagation_MD
      mask init:
      | DblOver = 0;
      mask TypeOptions PropDataTypeMode: Simulink:masks:SpecifyViaDialog | Simulink:masks:InheritViaPropagationRule
      mask Callback PropDataTypeMode: fixptdialog(gcbh)
      mask Callback PropDataType: fixptdialog(gcbh)
      mask TypeOptions IfRefDouble: Simulink:masks:double | Simulink:masks:single
      mask TypeOptions IfRefSingle: Simulink:masks:double | Simulink:masks:single
      mask TypeOptions IsSigned: Simulink:masks:IsSigned1 | Simulink:masks:IsSigned2 | Simulink:masks:IsSigned1OrIsSigned2 | Simulink:masks:TRUE | Simulink:masks:FALSE
      mask TypeOptions NumBitsBase: NumBits1 | NumBits2 | max([NumBits1 NumBits2]) | min([NumBits1 NumBits2]) | NumBits1+NumBits2
      mask TypeOptions PropScalingMode: Simulink:masks:SpecifyViaDialog | Simulink:masks:InheritViaPropagationRule | Simulink:masks:ObtainViaBestPrecision
      mask Callback PropScalingMode: fixptdialog(gcbh)
      mask TypeOptions SlopeBase: Slope1 | Slope2 | max([Slope1 Slope2]) | min([Slope1 Slope2]) | Slope1*Slope2 | Slope1/Slope2 | PosRange1 | PosRange2 | max([PosRange1 PosRange2]) | min([PosRange1 PosRange2]) | PosRange1*PosRange2 | PosRange1/PosRange2
      mask TypeOptions BiasBase: Bias1 | Bias2 | max([Bias1 Bias2]) | min([Bias1 Bias2]) | Bias1*Bias2 | Bias1/Bias2 | Bias1+Bias2 | Bias1-Bias2
      mask Display:
      | port_label('Input',1,'Ref1');
      | port_label('Input',2,'Ref2');
      | port_label('Input',3,'Prop');
  LowerRelop1 : RelationalOperator  DisableCoverage=on  Operator=>  OutDataTypeStr=boolean  RndMeth=Nearest
  Switch : Switch  Criteria=u2 ~= 0  OutDataTypeStr=Inherit: Inherit via back propagation  ZeroCross=off
  Switch2 : Switch  Criteria=u2 ~= 0  OutMin=OutMin  OutMax=OutMax  OutDataTypeStr=Inherit: Inherit via back propagation  ZeroCross=off
  UpperRelop : RelationalOperator  DisableCoverage=on  Operator=<  OutDataTypeStr=boolean  RndMeth=Nearest
  y : Outport  OutMin=OutMin  OutMax=OutMax
  wires:
  up/1 -> Switch2/1, LowerRelop1/2
  u/1 -> Data Type Propagation/2, Data Type Propagation/1, LowerRelop1/1, Switch/3, UpperRelop/1
  lo/1 -> Switch/1, UpperRelop/2
  Switch/1 -> Data Type Duplicate/2, Switch2/3, Data Type Propagation/3
  Switch2/1 -> Data Type Duplicate/1, y/1
  LowerRelop1/1 -> Switch2/2
  UpperRelop/1 -> Switch/2

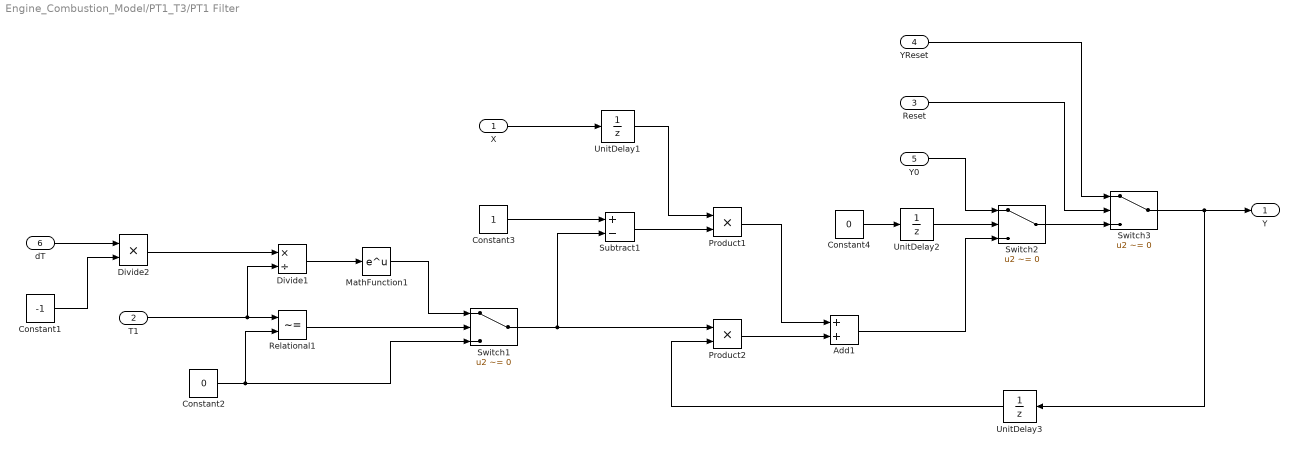
== system Engine_Combustion_Model/PT1_T3/PT1 Filter ==
  X : Inport
  T1 : Inport  Port=2
  Reset : Inport  Port=3
  YReset : Inport  Port=4
  Y0 : Inport  Port=5
  dT : Inport  Port=6
  Add1 : Sum
  Constant1 : Constant  Value=-1
  Constant2 : Constant  Value=0
  Constant3 : Constant
  Constant4 : Constant  Value=0
  Divide1 : Product  Inputs=*/
  Divide2 : Product  Inputs=**
  MathFunction1 : Math  SaturateOnIntegerOverflow=on
  Product1 : Product  RndMeth=Zero
  Product2 : Product  RndMeth=Zero
  Relational1 : RelationalOperator  Operator=~=  OutDataTypeStr=boolean  RndMeth=Nearest
  Subtract1 : Sum  Inputs=+-
  Switch1 : Switch  Criteria=u2 ~= 0
  Switch2 : Switch  Criteria=u2 ~= 0
  Switch3 : Switch  Criteria=u2 ~= 0
  UnitDelay1 : UnitDelay  SampleTime=-1
  UnitDelay2 : UnitDelay  InitialCondition=1  SampleTime=-1
  UnitDelay3 : UnitDelay  SampleTime=-1
  Y : Outport
  wires:
  Constant1/1 -> Divide2/2
  T1/1 -> Divide1/2, Relational1/1
  Divide2/1 -> Divide1/1
  Divide1/1 -> MathFunction1/1
  Constant3/1 -> Subtract1/1
  X/1 -> UnitDelay1/1
  UnitDelay1/1 -> Product1/1
  Subtract1/1 -> Product1/2
  Product1/1 -> Add1/1
  Product2/1 -> Add1/2
  Switch1/1 -> Subtract1/2, Product2/1
  UnitDelay3/1 -> Product2/2
  Reset/1 -> Switch3/2
  YReset/1 -> Switch3/1
  Constant4/1 -> UnitDelay2/1
  UnitDelay2/1 -> Switch2/2
  Y0/1 -> Switch2/1
  Switch3/1 -> UnitDelay3/1, Y/1
  Add1/1 -> Switch2/3
  Switch2/1 -> Switch3/3
  Relational1/1 -> Switch1/2
  MathFunction1/1 -> Switch1/1
  Constant2/1 -> Switch1/3, Relational1/2
  dT/1 -> Divide2/1

== system Engine_Combustion_Model/PT1_T3/Saturation Dynamic ==
  up : Inport
  u : Inport  Port=2
  lo : Inport  Port=3
  Data Type Duplicate : DataTypeDuplicate  DisableCoverage=on
  Data Type Propagation : S-Function  FunctionName=sfix_dtprop  Parameters=14,PropDataTypeMode,(getdatatypespecs(PropDataType,PropScaling,DblOver,0, 0, PropDataTypeMode, PropScalingMode)),IfRefDouble,IfRefSingle,IsSigned,NumBitsBase,NumBitsMult,NumBitsAdd,(sort(reshape(round(NumBitsAllowFinal), prod(size(NumBitsAllowFinal)),1))),PropScalingMode,ValuesUsedBestPrec,SlopeBase,SlopeMult,SlopeAdd,BiasBase,BiasMult,BiasAdd,DblOver  SFunctionDeploymentMode=off  EnableBusSupport=off  mask(Data Type Propagation){PropDataTypeMode=Inherit via propagation rule, PropDataType=fixdt(1, 16), IfRefDouble=double, IfRefSingle=single, IsSigned=IsSigned1, NumBitsBase=NumBits1, NumBitsMult=1, NumBitsAdd=0, NumBitsAllowFinal=1:128, PropScalingMode=Inherit via propagation rule, PropScaling=2^-10, ValuesUsedBestPrec=[5 -7], SlopeBase=Slope1, SlopeMult=1, SlopeAdd=0, BiasBase=Bias1, BiasMult=1, BiasAdd=0}
      mask prompts: PropDataTypeMode "Simulink:masks:x1PropagatedDataType_MP"; PropDataType "Simulink:masks:x11PropagatedDataTypeegFixdt116Fixdtsingle_MP"; IfRefDouble "Simulink:masks:x11IfAnyReferenceInputIsDoubleOutputIs_MP"; IfRefSingle "Simulink:masks:x12IfAnyReferenceInputIsSingleOutputIs_MP"; IsSigned "Simulink:masks:x13IsSigned_MP"; NumBitsBase "Simulink:masks:x141NumberofBitsBase_MP"; NumBitsMult "Simulink:masks:x142NumberofBitsMultiplicativeAdjustment_MP"; NumBitsAdd "Simulink:masks:x143NumberofBitsAdditiveAdjustment_MP"; NumBitsAllowFinal "Simulink:masks:x144NumberofBitsAllowableFinalValues_MP"; PropScalingMode "Simulink:masks:x2PropagatedScaling_MP"; PropScaling "Simulink:masks:x21PropagatedScalingSlopeEg29OrSlopeBiasEg1253_MP"; ValuesUsedBestPrec "Simulink:masks:x21ValuesUsedToDetermineBestPrecisionScaling_MP"; SlopeBase "Simulink:masks:x211SlopeBase_MP"; SlopeMult "Simulink:masks:x212SlopeMultiplicativeAdjustment_MP"; SlopeAdd "Simulink:masks:x213SlopeAdditiveAdjustment_MP"; BiasBase "Simulink:masks:x221BiasBase_MP"; BiasMult "Simulink:masks:x222BiasMultiplicativeAdjustment_MP"; BiasAdd "Simulink:masks:x223BiasAdditiveAdjustment_MP"
      mask help: Simulink:masks:DataTypePropagation_MD
      mask init:
      | DblOver = 0;
      mask TypeOptions PropDataTypeMode: Simulink:masks:SpecifyViaDialog | Simulink:masks:InheritViaPropagationRule
      mask Callback PropDataTypeMode: fixptdialog(gcbh)
      mask Callback PropDataType: fixptdialog(gcbh)
      mask TypeOptions IfRefDouble: Simulink:masks:double | Simulink:masks:single
      mask TypeOptions IfRefSingle: Simulink:masks:double | Simulink:masks:single
      mask TypeOptions IsSigned: Simulink:masks:IsSigned1 | Simulink:masks:IsSigned2 | Simulink:masks:IsSigned1OrIsSigned2 | Simulink:masks:TRUE | Simulink:masks:FALSE
      mask TypeOptions NumBitsBase: NumBits1 | NumBits2 | max([NumBits1 NumBits2]) | min([NumBits1 NumBits2]) | NumBits1+NumBits2
      mask TypeOptions PropScalingMode: Simulink:masks:SpecifyViaDialog | Simulink:masks:InheritViaPropagationRule | Simulink:masks:ObtainViaBestPrecision
      mask Callback PropScalingMode: fixptdialog(gcbh)
      mask TypeOptions SlopeBase: Slope1 | Slope2 | max([Slope1 Slope2]) | min([Slope1 Slope2]) | Slope1*Slope2 | Slope1/Slope2 | PosRange1 | PosRange2 | max([PosRange1 PosRange2]) | min([PosRange1 PosRange2]) | PosRange1*PosRange2 | PosRange1/PosRange2
      mask TypeOptions BiasBase: Bias1 | Bias2 | max([Bias1 Bias2]) | min([Bias1 Bias2]) | Bias1*Bias2 | Bias1/Bias2 | Bias1+Bias2 | Bias1-Bias2
      mask Display:
      | port_label('Input',1,'Ref1');
      | port_label('Input',2,'Ref2');
      | port_label('Input',3,'Prop');
  LowerRelop1 : RelationalOperator  DisableCoverage=on  Operator=>  OutDataTypeStr=boolean  RndMeth=Nearest
  Switch : Switch  Criteria=u2 ~= 0  OutDataTypeStr=Inherit: Inherit via back propagation  ZeroCross=off
  Switch2 : Switch  Criteria=u2 ~= 0  OutMin=OutMin  OutMax=OutMax  OutDataTypeStr=Inherit: Inherit via back propagation  ZeroCross=off
  UpperRelop : RelationalOperator  DisableCoverage=on  Operator=<  OutDataTypeStr=boolean  RndMeth=Nearest
  y : Outport  OutMin=OutMin  OutMax=OutMax
  wires:
  UpperRelop/1 -> Switch/2
  LowerRelop1/1 -> Switch2/2
  Switch2/1 -> y/1, Data Type Duplicate/1
  Switch/1 -> Data Type Propagation/3, Switch2/3, Data Type Duplicate/2
  lo/1 -> UpperRelop/2, Switch/1
  u/1 -> UpperRelop/1, Switch/3, LowerRelop1/1, Data Type Propagation/1, Data Type Propagation/2
  up/1 -> LowerRelop1/2, Switch2/1

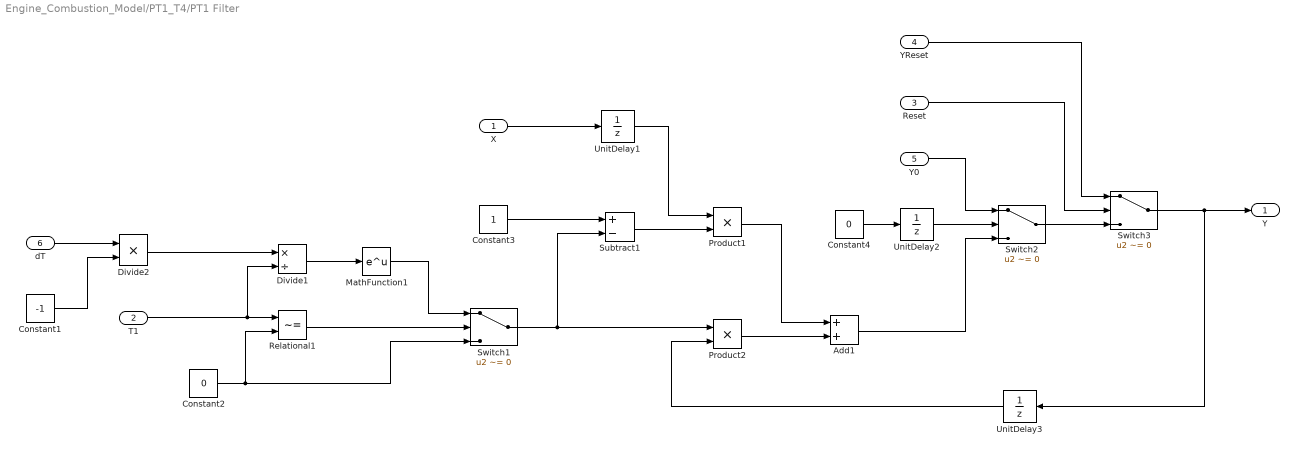
== system Engine_Combustion_Model/PT1_T4/PT1 Filter ==
  X : Inport
  T1 : Inport  Port=2
  Reset : Inport  Port=3
  YReset : Inport  Port=4
  Y0 : Inport  Port=5
  dT : Inport  Port=6
  Add1 : Sum
  Constant1 : Constant  Value=-1
  Constant2 : Constant  Value=0
  Constant3 : Constant
  Constant4 : Constant  Value=0
  Divide1 : Product  Inputs=*/
  Divide2 : Product  Inputs=**
  MathFunction1 : Math  SaturateOnIntegerOverflow=on
  Product1 : Product  RndMeth=Zero
  Product2 : Product  RndMeth=Zero
  Relational1 : RelationalOperator  Operator=~=  OutDataTypeStr=boolean  RndMeth=Nearest
  Subtract1 : Sum  Inputs=+-
  Switch1 : Switch  Criteria=u2 ~= 0
  Switch2 : Switch  Criteria=u2 ~= 0
  Switch3 : Switch  Criteria=u2 ~= 0
  UnitDelay1 : UnitDelay  SampleTime=-1
  UnitDelay2 : UnitDelay  InitialCondition=1  SampleTime=-1
  UnitDelay3 : UnitDelay  SampleTime=-1
  Y : Outport
  wires:
  dT/1 -> Divide2/1
  Constant2/1 -> Relational1/2, Switch1/3
  MathFunction1/1 -> Switch1/1
  Relational1/1 -> Switch1/2
  Switch2/1 -> Switch3/3
  Add1/1 -> Switch2/3
  Switch3/1 -> Y/1, UnitDelay3/1
  Y0/1 -> Switch2/1
  UnitDelay2/1 -> Switch2/2
  Constant4/1 -> UnitDelay2/1
  YReset/1 -> Switch3/1
  Reset/1 -> Switch3/2
  UnitDelay3/1 -> Product2/2
  Switch1/1 -> Product2/1, Subtract1/2
  Product2/1 -> Add1/2
  Product1/1 -> Add1/1
  Subtract1/1 -> Product1/2
  UnitDelay1/1 -> Product1/1
  X/1 -> UnitDelay1/1
  Constant3/1 -> Subtract1/1
  Divide1/1 -> MathFunction1/1
  Divide2/1 -> Divide1/1
  T1/1 -> Relational1/1, Divide1/2
  Constant1/1 -> Divide2/2

== system Engine_Combustion_Model/PT1_T4/Saturation Dynamic ==
  up : Inport
  u : Inport  Port=2
  lo : Inport  Port=3
  Data Type Duplicate : DataTypeDuplicate  DisableCoverage=on
  Data Type Propagation : S-Function  FunctionName=sfix_dtprop  Parameters=14,PropDataTypeMode,(getdatatypespecs(PropDataType,PropScaling,DblOver,0, 0, PropDataTypeMode, PropScalingMode)),IfRefDouble,IfRefSingle,IsSigned,NumBitsBase,NumBitsMult,NumBitsAdd,(sort(reshape(round(NumBitsAllowFinal), prod(size(NumBitsAllowFinal)),1))),PropScalingMode,ValuesUsedBestPrec,SlopeBase,SlopeMult,SlopeAdd,BiasBase,BiasMult,BiasAdd,DblOver  SFunctionDeploymentMode=off  EnableBusSupport=off  mask(Data Type Propagation){PropDataTypeMode=Inherit via propagation rule, PropDataType=fixdt(1, 16), IfRefDouble=double, IfRefSingle=single, IsSigned=IsSigned1, NumBitsBase=NumBits1, NumBitsMult=1, NumBitsAdd=0, NumBitsAllowFinal=1:128, PropScalingMode=Inherit via propagation rule, PropScaling=2^-10, ValuesUsedBestPrec=[5 -7], SlopeBase=Slope1, SlopeMult=1, SlopeAdd=0, BiasBase=Bias1, BiasMult=1, BiasAdd=0}
      mask prompts: PropDataTypeMode "Simulink:masks:x1PropagatedDataType_MP"; PropDataType "Simulink:masks:x11PropagatedDataTypeegFixdt116Fixdtsingle_MP"; IfRefDouble "Simulink:masks:x11IfAnyReferenceInputIsDoubleOutputIs_MP"; IfRefSingle "Simulink:masks:x12IfAnyReferenceInputIsSingleOutputIs_MP"; IsSigned "Simulink:masks:x13IsSigned_MP"; NumBitsBase "Simulink:masks:x141NumberofBitsBase_MP"; NumBitsMult "Simulink:masks:x142NumberofBitsMultiplicativeAdjustment_MP"; NumBitsAdd "Simulink:masks:x143NumberofBitsAdditiveAdjustment_MP"; NumBitsAllowFinal "Simulink:masks:x144NumberofBitsAllowableFinalValues_MP"; PropScalingMode "Simulink:masks:x2PropagatedScaling_MP"; PropScaling "Simulink:masks:x21PropagatedScalingSlopeEg29OrSlopeBiasEg1253_MP"; ValuesUsedBestPrec "Simulink:masks:x21ValuesUsedToDetermineBestPrecisionScaling_MP"; SlopeBase "Simulink:masks:x211SlopeBase_MP"; SlopeMult "Simulink:masks:x212SlopeMultiplicativeAdjustment_MP"; SlopeAdd "Simulink:masks:x213SlopeAdditiveAdjustment_MP"; BiasBase "Simulink:masks:x221BiasBase_MP"; BiasMult "Simulink:masks:x222BiasMultiplicativeAdjustment_MP"; BiasAdd "Simulink:masks:x223BiasAdditiveAdjustment_MP"
      mask help: Simulink:masks:DataTypePropagation_MD
      mask init:
      | DblOver = 0;
      mask TypeOptions PropDataTypeMode: Simulink:masks:SpecifyViaDialog | Simulink:masks:InheritViaPropagationRule
      mask Callback PropDataTypeMode: fixptdialog(gcbh)
      mask Callback PropDataType: fixptdialog(gcbh)
      mask TypeOptions IfRefDouble: Simulink:masks:double | Simulink:masks:single
      mask TypeOptions IfRefSingle: Simulink:masks:double | Simulink:masks:single
      mask TypeOptions IsSigned: Simulink:masks:IsSigned1 | Simulink:masks:IsSigned2 | Simulink:masks:IsSigned1OrIsSigned2 | Simulink:masks:TRUE | Simulink:masks:FALSE
      mask TypeOptions NumBitsBase: NumBits1 | NumBits2 | max([NumBits1 NumBits2]) | min([NumBits1 NumBits2]) | NumBits1+NumBits2
      mask TypeOptions PropScalingMode: Simulink:masks:SpecifyViaDialog | Simulink:masks:InheritViaPropagationRule | Simulink:masks:ObtainViaBestPrecision
      mask Callback PropScalingMode: fixptdialog(gcbh)
      mask TypeOptions SlopeBase: Slope1 | Slope2 | max([Slope1 Slope2]) | min([Slope1 Slope2]) | Slope1*Slope2 | Slope1/Slope2 | PosRange1 | PosRange2 | max([PosRange1 PosRange2]) | min([PosRange1 PosRange2]) | PosRange1*PosRange2 | PosRange1/PosRange2
      mask TypeOptions BiasBase: Bias1 | Bias2 | max([Bias1 Bias2]) | min([Bias1 Bias2]) | Bias1*Bias2 | Bias1/Bias2 | Bias1+Bias2 | Bias1-Bias2
      mask Display:
      | port_label('Input',1,'Ref1');
      | port_label('Input',2,'Ref2');
      | port_label('Input',3,'Prop');
  LowerRelop1 : RelationalOperator  DisableCoverage=on  Operator=>  OutDataTypeStr=boolean  RndMeth=Nearest
  Switch : Switch  Criteria=u2 ~= 0  OutDataTypeStr=Inherit: Inherit via back propagation  ZeroCross=off
  Switch2 : Switch  Criteria=u2 ~= 0  OutMin=OutMin  OutMax=OutMax  OutDataTypeStr=Inherit: Inherit via back propagation  ZeroCross=off
  UpperRelop : RelationalOperator  DisableCoverage=on  Operator=<  OutDataTypeStr=boolean  RndMeth=Nearest
  y : Outport  OutMin=OutMin  OutMax=OutMax
  wires:
  up/1 -> Switch2/1, LowerRelop1/2
  u/1 -> Data Type Propagation/2, Data Type Propagation/1, LowerRelop1/1, Switch/3, UpperRelop/1
  lo/1 -> Switch/1, UpperRelop/2
  Switch/1 -> Data Type Duplicate/2, Switch2/3, Data Type Propagation/3
  Switch2/1 -> Data Type Duplicate/1, y/1
  LowerRelop1/1 -> Switch2/2
  UpperRelop/1 -> Switch/2

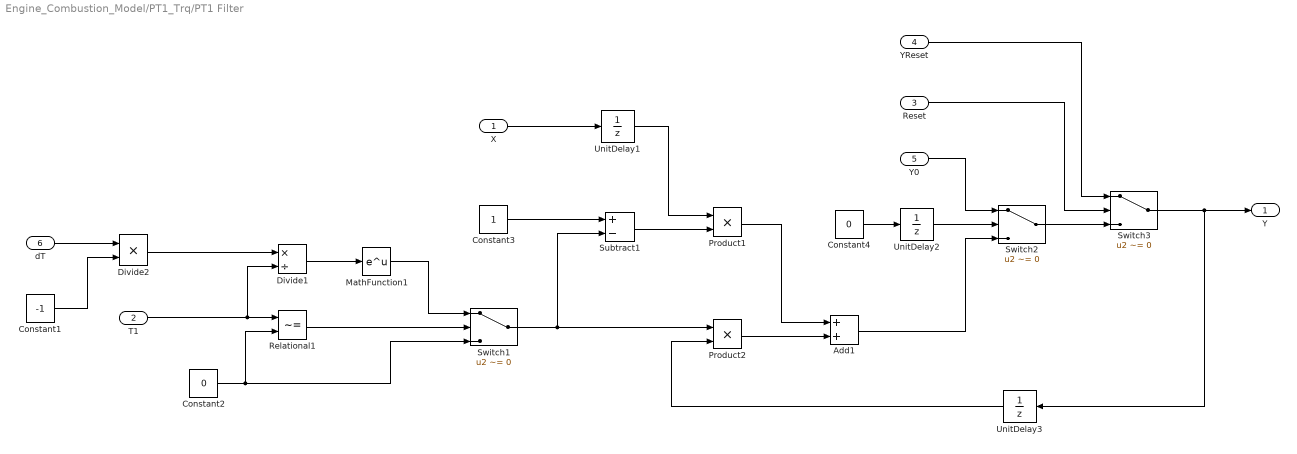
== system Engine_Combustion_Model/PT1_Trq/PT1 Filter ==
  X : Inport
  T1 : Inport  Port=2
  Reset : Inport  Port=3
  YReset : Inport  Port=4
  Y0 : Inport  Port=5
  dT : Inport  Port=6
  Add1 : Sum
  Constant1 : Constant  Value=-1
  Constant2 : Constant  Value=0
  Constant3 : Constant
  Constant4 : Constant  Value=0
  Divide1 : Product  Inputs=*/
  Divide2 : Product  Inputs=**
  MathFunction1 : Math  SaturateOnIntegerOverflow=on
  Product1 : Product  RndMeth=Zero
  Product2 : Product  RndMeth=Zero
  Relational1 : RelationalOperator  Operator=~=  OutDataTypeStr=boolean  RndMeth=Nearest
  Subtract1 : Sum  Inputs=+-
  Switch1 : Switch  Criteria=u2 ~= 0
  Switch2 : Switch  Criteria=u2 ~= 0
  Switch3 : Switch  Criteria=u2 ~= 0
  UnitDelay1 : UnitDelay  SampleTime=-1
  UnitDelay2 : UnitDelay  InitialCondition=1  SampleTime=-1
  UnitDelay3 : UnitDelay  SampleTime=-1
  Y : Outport
  wires:
  Constant1/1 -> Divide2/2
  T1/1 -> Divide1/2, Relational1/1
  Divide2/1 -> Divide1/1
  Divide1/1 -> MathFunction1/1
  Constant3/1 -> Subtract1/1
  X/1 -> UnitDelay1/1
  UnitDelay1/1 -> Product1/1
  Subtract1/1 -> Product1/2
  Product1/1 -> Add1/1
  Product2/1 -> Add1/2
  Switch1/1 -> Subtract1/2, Product2/1
  UnitDelay3/1 -> Product2/2
  Reset/1 -> Switch3/2
  YReset/1 -> Switch3/1
  Constant4/1 -> UnitDelay2/1
  UnitDelay2/1 -> Switch2/2
  Y0/1 -> Switch2/1
  Switch3/1 -> UnitDelay3/1, Y/1
  Add1/1 -> Switch2/3
  Switch2/1 -> Switch3/3
  Relational1/1 -> Switch1/2
  MathFunction1/1 -> Switch1/1
  Constant2/1 -> Switch1/3, Relational1/2
  dT/1 -> Divide2/1
